simulink model "model_induction_motor_v1"  (R2017b)
settings: Solver=VariableStepAuto  StartTime=0.0  StopTime=15  MaxStep=1e-4  RelTol=1e-3
libraries: powerlib x6
settings Model: SimulationMode=accelerator  Creator=proso  LastModifiedBy=proso

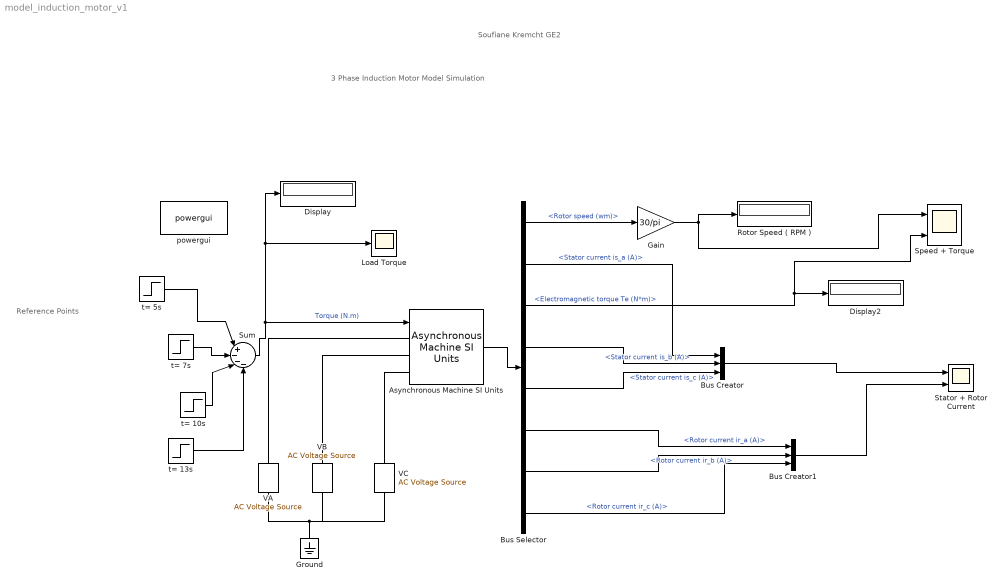
== system model_induction_motor_v1 ==
  note: Soufiane Kremcht GE2
  note: Reference Points
  note: 3 Phase Induction Motor Model Simulation
  Asynchronous Machine SI Units : powerlib/Machines/Asynchronous Machine SI Units  RotorType=Squirrel-cage  PresetModel="15:  5.4 HP (4KW)   400 V  50Hz 1430 RPM"  MechanicalLoad=Torque Tm  ShowDetailedParameters=on  ReferenceFrame=Rotor  Units=SI  MeasurementBus=off  NominalParameters=[4000 400 50]  Stator=[1.405 0.005839]  Rotor=[1.395 0.005839]  Cage1=[1.543 0.006067]  Cage2=[3.309 0.005654]  Lm=0.1722  Mechanical=[0.0131 0.002985 2]  PolePairs=2  InitialConditions=[1 0 0 0 0 0 0 0]  SimulateSaturation=off  Saturation=[14.03593122, 27.81365428, 53.79336849, 72.68890987, 97.98006896, 148.6815601, 215.7428561, 302.9841135, 428.7778367 ; 230, 322, 414, 460, 506, 552, 598, 644, 690]  LoadFlowParameters=1492000  TsPowergui=0  TsBlock=-1  IterativeModel=Trapezoidal non iterative  IterativeDiscreteModel=Trapezoidal non iterative  Pmec=1.492e+006
  Bus Creator : BusCreator  Inputs=3
  Bus Creator1 : BusCreator  Inputs=3
  Bus Selector : BusSelector  OutputSignals=Mechanical.Rotor speed (wm),Stator measurements.Stator current is_a (A),Mechanical.Electromagnetic torque Te (N*m),Stator measurements.Stator current is_b (A),Stator measurements.Stator current is_c (A),Rotor measurements.Rotor current ir_a (A),Rotor measurements.Rotor current ir_b (A),Rotor measurements.Rotor current ir_c (A)
  Display : Display
  Display2 : Display
  Gain : Gain  Gain=30/pi
  Ground : powerlib/Elements/Ground  LConnTagsString=a
  Load Torque : Scope
  Rotor Speed ( RPM ) : Display
  Speed + Torque : Scope  NumInputPorts=2
  Stator + Rotor Current : Scope  NumInputPorts=2
  Sum : Sum  Inputs=|+---
  VA : powerlib/Electrical Sources/AC Voltage Source  Amplitude=380  Phase=0  Frequency=50  SampleTime=0  Measurements=None  BusType=swing  Pref=10e3  Qref=0  Qmin=-inf  Qmax=+inf
  VB : powerlib/Electrical Sources/AC Voltage Source  Amplitude=380  Phase=-120  Frequency=50  SampleTime=0  Measurements=None  BusType=swing  Pref=10e3  Qref=0  Qmin=-inf  Qmax=+inf
  VC : powerlib/Electrical Sources/AC Voltage Source  Amplitude=380  Phase=120  Frequency=50  SampleTime=0  Measurements=None  BusType=swing  Pref=10e3  Qref=0  Qmin=-inf  Qmax=+inf
  powergui : powerlib/powergui  Priority=1  SimulationMode=Continuous  SampleTime=50e-6  frequency=60  Iterations=50  frequencyindice=50  Pbase=100e6  ErrMax=1e-4  UnitsV=kV  UnitsW=MW  buscounter=0  FunctionMessages=off  echomessages=off  EnableUseOfTLC=off  CurrentSourceSwitches=off  DisableSnubberDevices=off  DisableRonSwitches=off  DisableVfSwitches=off  DisplayEquations=off  SolverType=Tustin/Backward Euler (TBE)  Interpol=off  ExternalGateDelay=off  methode=off  Ts=100  x0status=blocks  SPID=on  SwTol=0  HookPort=off  RestoreLinks=warning  ResistiveCurrentMeasurement=off  Frange=[0:2:500]  Ylog=off  Xlog=on  ShowGrid=off  save=off  variable=ZData  structure=0  ZoomFFT=off  StartTime=0.0  cycles=1  DisplayStyle=1  fundamental=60  FreqAxis=off  MaxFrequency=1000  frequencyindicesteady=1  RmsSteady=1  display=off
  t= 10s : Step  Time=10  After=6.68  SampleTime=0
  t= 13s : Step  Time=13  After=6.68  SampleTime=0
  t= 5s : Step  Time=3  After=26.5  SampleTime=0
  t= 7s : Step  Time=5  After=13  SampleTime=0
  wires:
  t= 5s/1 -> Sum/1
  t= 7s/1 -> Sum/2
  t= 10s/1 -> Sum/3
  t= 13s/1 -> Sum/4
  Sum/1 -> Load Torque/1, Display/1, Asynchronous Machine SI Units/1  "Torque (N.m)"
  Asynchronous Machine SI Units/1 -> Bus Selector/1
  Bus Selector/1 -> Gain/1  "<Rotor speed (wm)>"
  Gain/1 -> Speed + Torque/1, Rotor Speed ( RPM )/1
  Bus Creator/1 -> Stator + Rotor Current/1
  Bus Creator1/1 -> Stator + Rotor Current/2
  Bus Selector/3 -> Speed + Torque/2, Display2/1  "<Electromagnetic torque Te (N*m)>"
  Bus Selector/2 -> Bus Creator/1  "<Stator current is_a (A)>"
  Bus Selector/4 -> Bus Creator/2  "<Stator current is_b (A)>"
  Bus Selector/5 -> Bus Creator/3  "<Stator current is_c (A)>"
  Bus Selector/6 -> Bus Creator1/1  "<Rotor current ir_a (A)>"
  Bus Selector/7 -> Bus Creator1/2  "<Rotor current ir_b (A)>"
  Bus Selector/8 -> Bus Creator1/3  "<Rotor current ir_c (A)>"
  connections:
  VA/LConn1 -- VC/LConn1 -- VB/LConn1 -- Ground/LConn1
  VA/RConn1 -- Asynchronous Machine SI Units/LConn1
  VB/RConn1 -- Asynchronous Machine SI Units/LConn2
  VC/RConn1 -- Asynchronous Machine SI Units/LConn3
